simulink model "lazoAbierto"  (R2018a)
settings: Solver=VariableStepAuto  StartTime=0.0  StopTime=25  RelTol=1e-3
values from neighbouring files (symbols this model uses):
  C = 2267    [paramsLinealizado.m]
  H_l = 1.05    [paramsLinealizado.m]
  n0_S = 1322    [paramsLinealizado.m]
  P_cp = 1924    [paramsLinealizado.m]
  Tinit = 260    [paramsLinealizado.m]
libraries: simulink x11
settings Model: Creator=wenap  LastModifiedBy=chris
settings DataIOCC: ReturnWorkspaceOutputs=on
settings SFSimCC: SimUseLocalCustomCode=on
settings RTWCC: RTWUseLocalCustomCode=on

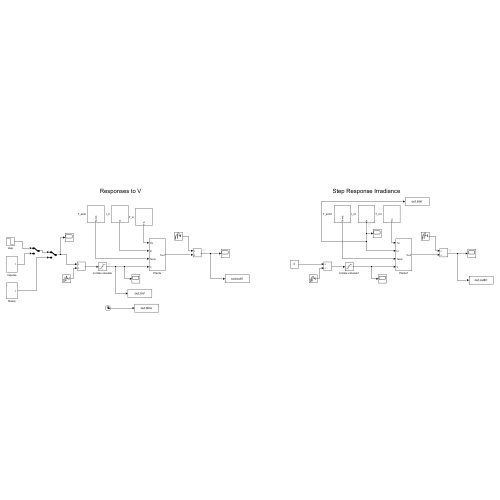
[thumbnail: Simulink's stored preview of the top-level diagram]
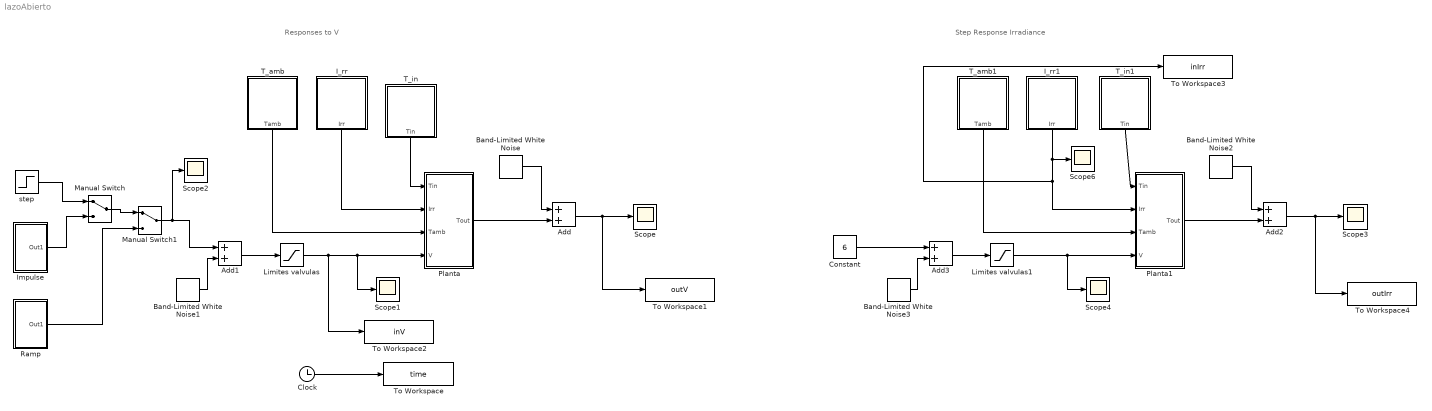
== system lazoAbierto ==
  note: Responses to V
  note: Step Response Irradiance
  Add{,1..3} (4 alike) : Sum
  Band-Limited White Noise : simulink/Sources/Band-Limited White Noise  Cov=[0.0001]  Ts=0.5  seed=[23341]
  Band-Limited White Noise1 : simulink/Sources/Band-Limited White Noise  Cov=[0.0001]  Ts=0.5  seed=[0]
  Band-Limited White Noise2 : simulink/Sources/Band-Limited White Noise  Cov=[0.0001]  Ts=0.5  seed=[23341]
  Band-Limited White Noise3 : simulink/Sources/Band-Limited White Noise  Cov=[0.0001]  Ts=0.5  seed=[0]
  Clock : Clock
  Constant : Constant  Value=6
  I_rr : Subsystem
  I_rr1 : Subsystem
  Impulse : Subsystem
  Limites valvulas : Saturate  UpperLimit=12  LowerLimit=2
  Limites valvulas1 : Saturate  UpperLimit=12  LowerLimit=2
  Manual Switch : ManualSwitch
  Manual Switch1 : ManualSwitch
  Planta : Subsystem
  Planta1 : Subsystem
  Ramp : Subsystem
  Scope{,1..4,6} (6 alike) : Scope
  T_amb : Subsystem
  T_amb1 : Subsystem
  T_in : Subsystem
  T_in1 : Subsystem
  To Workspace : ToWorkspace  VariableName=time  SampleTime=-1
  To Workspace1 : ToWorkspace  VariableName=outV  SaveFormat=Timeseries  SampleTime=-1
  To Workspace2 : ToWorkspace  VariableName=inV  SaveFormat=Timeseries  SampleTime=-1
  To Workspace3 : ToWorkspace  VariableName=inIrr  SaveFormat=Timeseries  SampleTime=-1
  To Workspace4 : ToWorkspace  VariableName=outIrr  SaveFormat=Timeseries  SampleTime=-1
  step : Step  Time=5  Before=8  After=7  SampleTime=0
  wires:
  T_in/1(Tin) -> Planta/1(Tin)
  I_rr/1(Irr) -> Planta/2(Irr)
  T_amb/1(Tamb) -> Planta/3(Tamb)
  Add/1 -> To Workspace1/1, Scope/1
  Planta/1(Tout) -> Add/2
  Band-Limited White Noise/1 -> Add/1
  Band-Limited White Noise1/1 -> Add1/2
  Limites valvulas/1 -> To Workspace2/1, Scope1/1, Planta/4(V)
  Add1/1 -> Limites valvulas/1
  Clock/1 -> To Workspace/1
  Manual Switch/1 -> Manual Switch1/1
  step/1 -> Manual Switch/1
  Impulse/1(Out1) -> Manual Switch/2
  Ramp/1(Out1) -> Manual Switch1/2
  Manual Switch1/1 -> Scope2/1, Add1/1
  T_in1/1(Tin) -> Planta1/1(Tin)
  Add3/1 -> Limites valvulas1/1
  Add2/1 -> To Workspace4/1, Scope3/1
  Planta1/1(Tout) -> Add2/2
  I_rr1/1(Irr) -> Scope6/1, Planta1/2(Irr), To Workspace3/1
  Limites valvulas1/1 -> Scope4/1, Planta1/4(V)
  Band-Limited White Noise2/1 -> Add2/1
  Band-Limited White Noise3/1 -> Add3/2
  T_amb1/1(Tamb) -> Planta1/3(Tamb)
  Constant/1 -> Add3/1

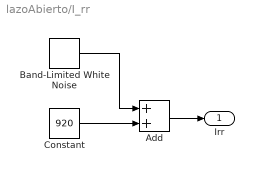
== system lazoAbierto/I_rr ==
  Add : Sum
  Band-Limited White Noise : simulink/Sources/Band-Limited White Noise  Cov=[0.0001]  Ts=1  seed=[2]
  Constant : Constant  Value=920
  Irr : Outport
  wires:
  Constant/1 -> Add/2
  Add/1 -> Irr/1
  Band-Limited White Noise/1 -> Add/1

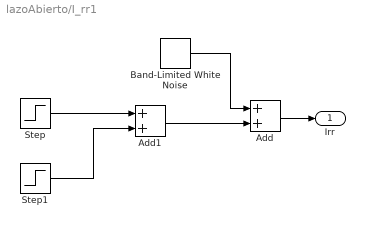
== system lazoAbierto/I_rr1 ==
  Add : Sum
  Add1 : Sum
  Band-Limited White Noise : simulink/Sources/Band-Limited White Noise  Cov=[0.0001]  Ts=1  seed=[2]
  Step : Step  Time=5  Before=840  After=600  SampleTime=0
  Step1 : Step  Time=15  After=200  SampleTime=0
  Irr : Outport
  wires:
  Add/1 -> Irr/1
  Band-Limited White Noise/1 -> Add/1
  Add1/1 -> Add/2
  Step/1 -> Add1/1
  Step1/1 -> Add1/2

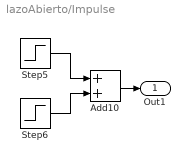
== system lazoAbierto/Impulse ==
  Add10 : Sum
  Step5 : Step  Time=5  Before=2  After=12  SampleTime=0
  Step6 : Step  Time=8  After=-10  SampleTime=0
  Out1 : Outport
  wires:
  Step5/1 -> Add10/1
  Step6/1 -> Add10/2
  Add10/1 -> Out1/1

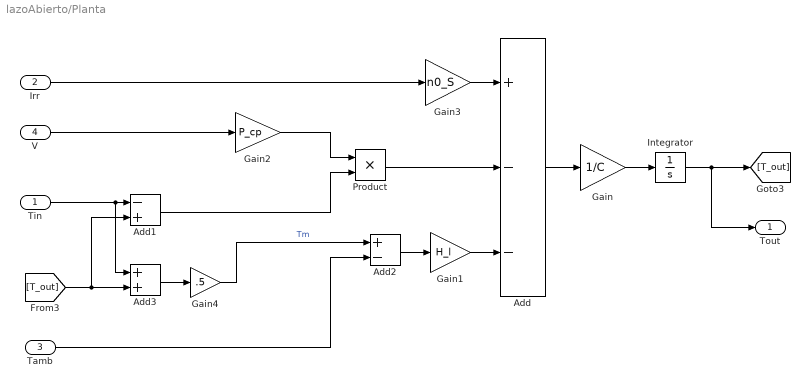
== system lazoAbierto/Planta ==
  Tin : Inport
  Irr : Inport  Port=2
  Tamb : Inport  Port=3
  V : Inport  Port=4
  Add : Sum  Inputs=+--
  Add1 : Sum  Inputs=-+
  Add2 : Sum  Inputs=+-
  Add3 : Sum
  Gain : Gain  Gain=1/C
  Gain1 : Gain  Gain=H_l
  Gain2 : Gain  Gain=P_cp
  Gain3 : Gain  Gain=n0_S
  Gain4 : Gain  Gain=.5
  Integrator : Integrator  InitialCondition=Tinit
  Product : Product
  Tout : Outport
  wires:
  Gain2/1 -> Product/1
  Gain3/1 -> Add/1
  Add2/1 -> Gain1/1
  Add1/1 -> Product/2
  Gain/1 -> Integrator/1
  Integrator/1 -> Tout/1, [T_out]
  Add3/1 -> Gain4/1
  Tamb/1 -> Add2/2
  [T_out] -> Add3/2, Add1/2
  Tin/1 -> Add3/1, Add1/1
  Add/1 -> Gain/1
  Product/1 -> Add/2
  Gain1/1 -> Add/3
  Irr/1 -> Gain3/1
  Gain4/1 -> Add2/1  "Tm"
  V/1 -> Gain2/1

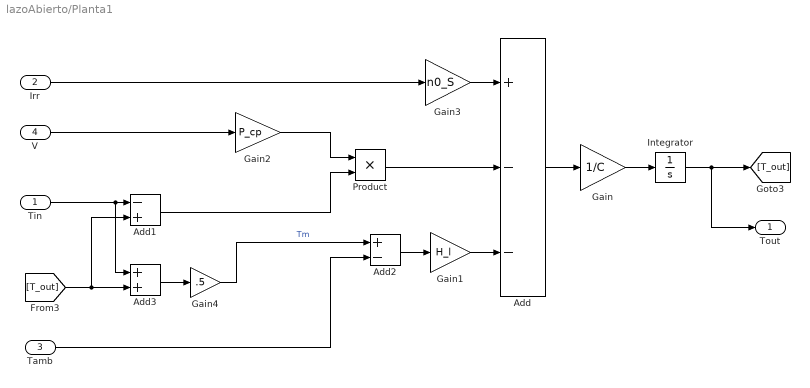
== system lazoAbierto/Planta1 ==
  Tin : Inport
  Irr : Inport  Port=2
  Tamb : Inport  Port=3
  V : Inport  Port=4
  Add : Sum  Inputs=+--
  Add1 : Sum  Inputs=-+
  Add2 : Sum  Inputs=+-
  Add3 : Sum
  Gain : Gain  Gain=1/C
  Gain1 : Gain  Gain=H_l
  Gain2 : Gain  Gain=P_cp
  Gain3 : Gain  Gain=n0_S
  Gain4 : Gain  Gain=.5
  Integrator : Integrator  InitialCondition=Tinit
  Product : Product
  Tout : Outport
  wires:
  Gain2/1 -> Product/1
  Gain3/1 -> Add/1
  Add2/1 -> Gain1/1
  Add1/1 -> Product/2
  Gain/1 -> Integrator/1
  Integrator/1 -> Tout/1, [T_out]
  Add3/1 -> Gain4/1
  Tamb/1 -> Add2/2
  [T_out] -> Add3/2, Add1/2
  Tin/1 -> Add3/1, Add1/1
  Add/1 -> Gain/1
  Product/1 -> Add/2
  Gain1/1 -> Add/3
  Irr/1 -> Gain3/1
  Gain4/1 -> Add2/1  "Tm"
  V/1 -> Gain2/1

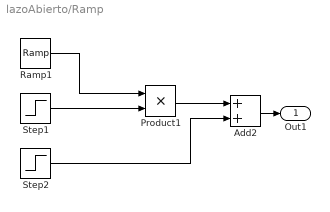
== system lazoAbierto/Ramp ==
  Add2 : Sum
  Product1 : Product
  Ramp1 : simulink/Sources/Ramp  slope=3.33  start=5  InitialOutput=2
  Step1 : Step  Time=8  Before=1  After=0  SampleTime=0
  Step2 : Step  Time=8  After=2  SampleTime=0
  Out1 : Outport
  wires:
  Product1/1 -> Add2/1
  Ramp1/1 -> Product1/1
  Step1/1 -> Product1/2
  Add2/1 -> Out1/1
  Step2/1 -> Add2/2

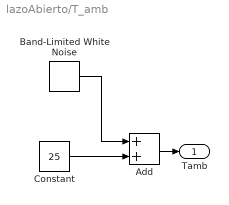
== system lazoAbierto/T_amb ==
  Add : Sum
  Band-Limited White Noise : simulink/Sources/Band-Limited White Noise  Cov=[0.0001]  Ts=0.1  seed=[1]
  Constant : Constant  Value=25
  Tamb : Outport
  wires:
  Constant/1 -> Add/2
  Add/1 -> Tamb/1
  Band-Limited White Noise/1 -> Add/1

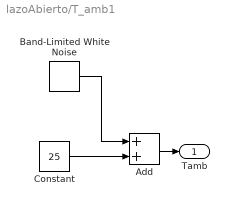
== system lazoAbierto/T_amb1 ==
  Add : Sum
  Band-Limited White Noise : simulink/Sources/Band-Limited White Noise  Cov=[0.0001]  Ts=0.1  seed=[1]
  Constant : Constant  Value=25
  Tamb : Outport
  wires:
  Constant/1 -> Add/2
  Add/1 -> Tamb/1
  Band-Limited White Noise/1 -> Add/1

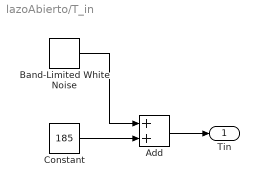
== system lazoAbierto/T_in ==
  Add : Sum
  Band-Limited White Noise : simulink/Sources/Band-Limited White Noise  Cov=[0.0001]  Ts=1  seed=[3]
  Constant : Constant  Value=185
  Tin : Outport
  wires:
  Add/1 -> Tin/1
  Constant/1 -> Add/2
  Band-Limited White Noise/1 -> Add/1

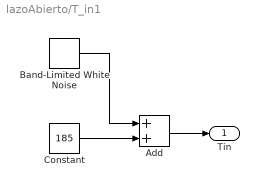
== system lazoAbierto/T_in1 ==
  Add : Sum
  Band-Limited White Noise : simulink/Sources/Band-Limited White Noise  Cov=[0.0001]  Ts=1  seed=[3]
  Constant : Constant  Value=185
  Tin : Outport
  wires:
  Add/1 -> Tin/1
  Constant/1 -> Add/2
  Band-Limited White Noise/1 -> Add/1
